simulink model "Lab5p3b"  (R2022a)
settings: Solver=ode3  StartTime=0.0  StopTime=Tmdl  FixedStep=T0/100  RelTol=1e-3
values from neighbouring files (symbols this model uses):
  ob =     [data.mat]
undefined symbols (not defined in the file or in its folder): spl, T0
libraries: fl_lib x22, nesl_utility x18
settings Model: Creator=Egor  LastModifiedBy=vardo

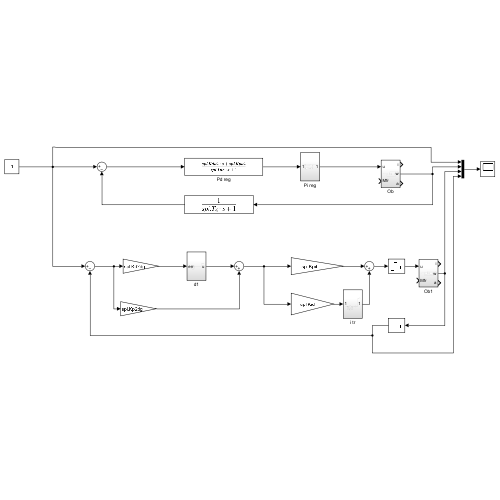
[thumbnail: Simulink's stored preview of the top-level diagram]
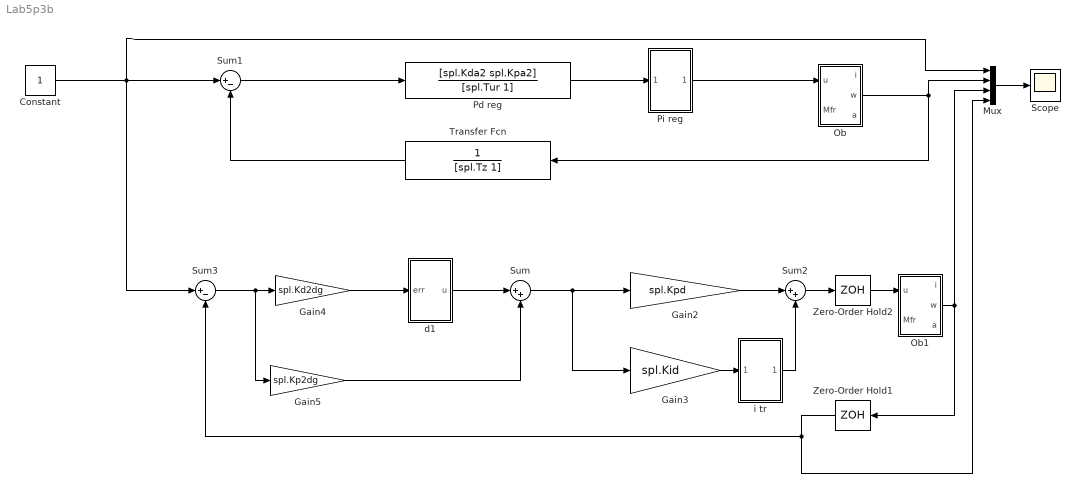
== system Lab5p3b ==
  Constant : Constant
  Gain2 : Gain  Gain=spl.Kpd
  Gain3 : Gain  Gain=spl.Kid
  Gain4 : Gain  Gain=spl.Kd2dg
  Gain5 : Gain  Gain=spl.Kp2dg
  Mux : Mux
  Ob : Subsystem
  Ob1 : Subsystem
  Pd reg : TransferFcn  Numerator=[spl.Kda2 spl.Kpa2]  Denominator=[spl.Tur 1]
  Pi reg : Subsystem
  Scope : Scope
  Sum : Sum  Inputs=|++
  Sum1 : Sum  Inputs=|+-
  Sum2 : Sum  Inputs=|++
  Sum3 : Sum  Inputs=|+-
  Transfer Fcn : TransferFcn  Denominator=[spl.Tz 1]
  Zero-Order Hold1 : ZeroOrderHold  SampleTime=T0
  Zero-Order Hold2 : ZeroOrderHold  SampleTime=T0
  d1 : Subsystem
  i tr : Subsystem
  wires:
  Mux/1 -> Scope/1
  Sum2/1 -> Zero-Order Hold2/1
  i tr/1(Out1) -> Sum2/2
  Gain2/1 -> Sum2/1
  Constant/1 -> Sum3/1, Mux/1, Sum1/1
  Ob1/2(w) -> Mux/3, Zero-Order Hold1/1
  Gain3/1 -> i tr/1(In1)
  Zero-Order Hold2/1 -> Ob1/1(u)
  Zero-Order Hold1/1 -> Mux/4, Sum3/2
  Ob/2(w) -> Transfer Fcn/1, Mux/2
  Sum1/1 -> Pd reg/1
  Pi reg/1(Out1) -> Ob/1(u)
  Pd reg/1 -> Pi reg/1(In1)
  d1/1(u) -> Sum/1
  Gain5/1 -> Sum/2
  Sum3/1 -> Gain5/1, Gain4/1
  Gain4/1 -> d1/1(err)
  Sum/1 -> Gain3/1, Gain2/1
  Transfer Fcn/1 -> Sum1/2

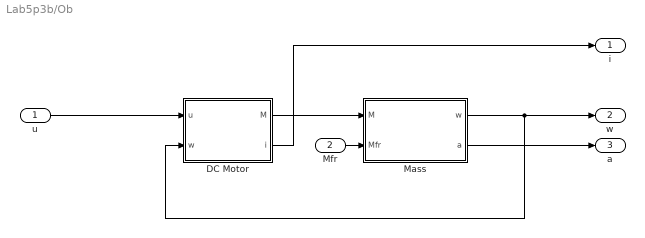
== system Lab5p3b/Ob ==
  u : Inport
  Mfr : Inport  Port=2
  DC Motor : Subsystem
  Mass : Subsystem
  i : Outport
  w : Outport  Port=2
  a : Outport  Port=3
  wires:
  Mass/2(a) -> a/1
  u/1 -> DC Motor/1(u)
  Mass/1(w) -> w/1, DC Motor/2(w)
  DC Motor/1(M) -> Mass/1(M)
  Mfr/1 -> Mass/2(Mfr)
  DC Motor/2(i) -> i/1

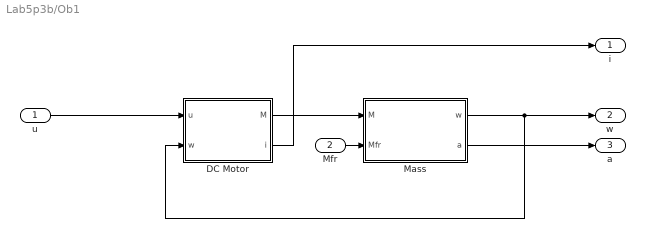
== system Lab5p3b/Ob1 ==
  u : Inport
  Mfr : Inport  Port=2
  DC Motor : Subsystem
  Mass : Subsystem
  i : Outport
  w : Outport  Port=2
  a : Outport  Port=3
  wires:
  Mass/2(a) -> a/1
  u/1 -> DC Motor/1(u)
  Mass/1(w) -> w/1, DC Motor/2(w)
  DC Motor/1(M) -> Mass/1(M)
  Mfr/1 -> Mass/2(Mfr)
  DC Motor/2(i) -> i/1

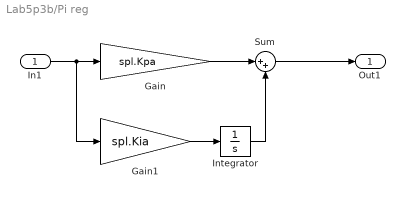
== system Lab5p3b/Pi reg ==
  In1 : Inport
  Gain : Gain  Gain=spl.Kpa
  Gain1 : Gain  Gain=spl.Kia
  Integrator : Integrator
  Sum : Sum  Inputs=|++
  Out1 : Outport
  wires:
  Gain1/1 -> Integrator/1
  In1/1 -> Gain1/1, Gain/1
  Integrator/1 -> Sum/2
  Gain/1 -> Sum/1
  Sum/1 -> Out1/1

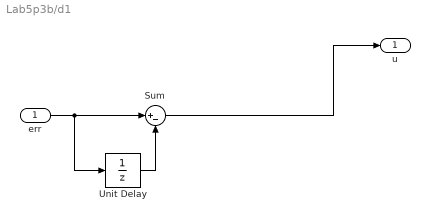
== system Lab5p3b/d1 ==
  err : Inport
  Sum : Sum  Inputs=|+-
  Unit Delay : UnitDelay  SampleTime=T0  HasFrameUpgradeWarning=on
  u : Outport
  wires:
  err/1 -> Unit Delay/1, Sum/1
  Unit Delay/1 -> Sum/2
  Sum/1 -> u/1

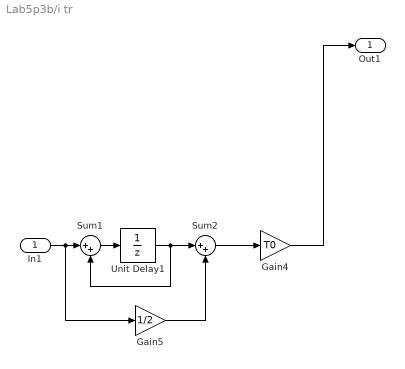
== system Lab5p3b/i tr ==
  In1 : Inport
  Gain4 : Gain  Gain=T0
  Gain5 : Gain  Gain=1/2
  Sum1 : Sum  Inputs=|++
  Sum2 : Sum  Inputs=|++
  Unit Delay1 : UnitDelay  SampleTime=-1  HasFrameUpgradeWarning=on
  Out1 : Outport
  wires:
  In1/1 -> Gain5/1, Sum1/1
  Sum1/1 -> Unit Delay1/1
  Gain5/1 -> Sum2/2
  Gain4/1 -> Out1/1
  Unit Delay1/1 -> Sum2/1, Sum1/2
  Sum2/1 -> Gain4/1

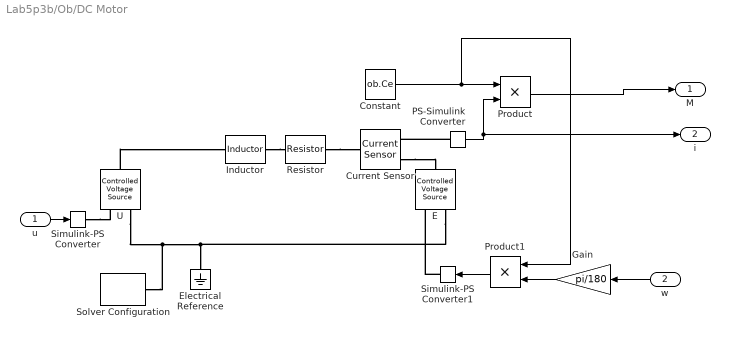
== system Lab5p3b/Ob/DC Motor ==
  u : Inport
  w : Inport  Port=2
  Constant : Constant  Value=ob.Ce
  Current Sensor : fl_lib/Electrical/Electrical Sensors/Current Sensor
      settings: SourceProductBaseCode=PW,SS,VE
  E : fl_lib/Electrical/Electrical Sources/Controlled Voltage Source
      settings: SourceProductBaseCode=PW,SS,VE
  Electrical Reference : fl_lib/Electrical/Electrical Elements/Electrical Reference
      settings: SourceProductBaseCode=PW,SS,VE
  Gain : Gain  Gain=pi/180
  Inductor : fl_lib/Electrical/Electrical Elements/Inductor  l=ob.L H  r=0 Ohm  g=1e-9 1/Ohm  i_specify=off  i_priority=None  i=0 A  i_nominal_specify=off  i_nominal_unit=A  i_nominal_value=1  v_specify=off  v_priority=None  v=0 V  v_nominal_specify=off  v_nominal_unit=V  v_nominal_value=1  i_L_specify=off  i_L_priority=High  i_L=0 A  i_L_nominal_specify=off  i_L_nominal_unit=A  i_L_nominal_value=1
      settings: SourceProductBaseCode=PW,SS,VE
  PS-Simulink Converter : nesl_utility/PS-Simulink Converter  PhysicalDomain=network_engine_domain  SubClassName=ps_output  LeftPortType=input  RightPortType=output  PseudoPeriodic=off  Frequencies=[]  VectorFormat=inherit  Unit=inherit  AffineConversion=off
      settings: SourceProductBaseCode=SS,PW,VE
  Product : Product
  Product1 : Product
  Resistor : fl_lib/Electrical/Electrical Elements/Resistor  R=ob.R Ohm  i_specify=off  i_priority=None  i=0 A  i_nominal_specify=off  i_nominal_unit=A  i_nominal_value=1  v_specify=off  v_priority=None  v=0 V  v_nominal_specify=off  v_nominal_unit=V  v_nominal_value=1
      settings: SourceProductBaseCode=PW,SS,VE
  Simulink-PS Converter : nesl_utility/Simulink-PS Converter  PhysicalDomain=network_engine_domain  SubClassName=ps_input  LeftPortType=input  RightPortType=output  PseudoPeriodic=off  Frequencies=[]  NoiseDistribution=none  NoiseParameters=[]  Unit=1  AffineConversion=off  FilteringAndDerivatives=provide  SimscapeFilterOrder=1  InputFilterTimeConstant=0.0001  UdotUserProvided=0
      settings: SourceProductBaseCode=SS,PW,VE
  Simulink-PS Converter1 : nesl_utility/Simulink-PS Converter  PhysicalDomain=network_engine_domain  SubClassName=ps_input  LeftPortType=input  RightPortType=output  PseudoPeriodic=off  Frequencies=[]  NoiseDistribution=none  NoiseParameters=[]  Unit=1  AffineConversion=off  FilteringAndDerivatives=provide  SimscapeFilterOrder=1  InputFilterTimeConstant=0.001  UdotUserProvided=0
      settings: SourceProductBaseCode=SS,PW,VE
  Solver Configuration : nesl_utility/Solver Configuration  PhysicalDomain=network_engine_domain  SubClassName=solver  LeftPortType=input  RightPortType=generic  Tones=[]  Harmonics=[]  SimulateNoise=off  Profile=off  UseLocalSampling=off  EnableSwitchedLinearOptims=on  FrequencyDomain=off  UseCCode=off  RelTol=0.001  AbsTol=0.001  MinStep=1e-09  ToWorkspace=off  RevertToSquareIcSolve=off  NumHomotopyIterations=100  PhasorMode=off  PhasorModeNumHarmonics=1  IndexReductionMethod=DerivativeReplacement  DoDC=off  ResidualTolerance=1e-09  UseLocalSolver=off  LocalSolverChoice=NE_BACKWARD_EULER_ADVANCER  LocalSolverSampleTime=0.001  DoFixedCost=off  MaxNonlinIter=3  MaxModeIter=2  ComputeImpulses=off  ImpulseIterations=2  LinearAlgebra=auto  LinearAlgebraNumThread=0  EquationFormulation=NE_TIME_EF  DelaysMemoryBudget=1024  AutomaticFiltering=on  FilteringTimeConstant=0.001  PartitionStorageMethod=AS_NEEDED  PartitionMemoryBudget=1024  PartitionMethod=ROBUST
      settings: SourceProductBaseCode=SS,PW,VE
  U : fl_lib/Electrical/Electrical Sources/Controlled Voltage Source
      settings: SourceProductBaseCode=PW,SS,VE
  M : Outport
  i : Outport  Port=2
  wires:
  PS-Simulink Converter/1 -> i/1, Product/2
  Product1/1 -> Simulink-PS Converter1/1
  Constant/1 -> Product1/1, Product/1
  Product/1 -> M/1
  u/1 -> Simulink-PS Converter/1
  w/1 -> Gain/1
  Gain/1 -> Product1/2
  connections:
  Simulink-PS Converter1/RConn1 -- E/RConn1
  Current Sensor/RConn2 -- E/LConn1
  U/LConn1 -- Inductor/LConn1
  U/RConn2 -- Solver Configuration/RConn1 -- E/RConn2 -- Electrical Reference/LConn1
  Resistor/RConn1 -- Current Sensor/LConn1
  Simulink-PS Converter/RConn1 -- U/RConn1
  PS-Simulink Converter/LConn1 -- Current Sensor/RConn1
  Inductor/RConn1 -- Resistor/LConn1

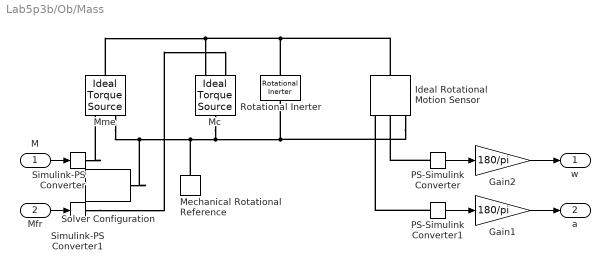
== system Lab5p3b/Ob/Mass ==
  M : Inport
  Mfr : Inport  Port=2
  Gain1 : Gain  Gain=180/pi
  Gain2 : Gain  Gain=180/pi
  Ideal Rotational Motion Sensor : fl_lib/Mechanical/Mechanical Sensors/Ideal Rotational Motion Sensor  wrap_angle=simscape.enum.onoff.off  offset=0 rad
      settings: SourceProductBaseCode=PW,SS,VE
  Mc : fl_lib/Mechanical/Mechanical Sources/Ideal Torque Source
      settings: SourceProductBaseCode=PW,SS,VE
  Mechanical Rotational Reference : fl_lib/Mechanical/Rotational Elements/Mechanical Rotational Reference
      settings: SourceProductBaseCode=PW,SS,VE
  Mme : fl_lib/Mechanical/Mechanical Sources/Ideal Torque Source
      settings: SourceProductBaseCode=PW,SS,VE
  PS-Simulink Converter : nesl_utility/PS-Simulink Converter  PhysicalDomain=network_engine_domain  SubClassName=ps_output  LeftPortType=input  RightPortType=output  PseudoPeriodic=off  Frequencies=[]  VectorFormat=inherit  Unit=inherit  AffineConversion=off
      settings: SourceProductBaseCode=SS,PW,VE
  PS-Simulink Converter1 : nesl_utility/PS-Simulink Converter  PhysicalDomain=network_engine_domain  SubClassName=ps_output  LeftPortType=input  RightPortType=output  PseudoPeriodic=off  Frequencies=[]  VectorFormat=inherit  Unit=inherit  AffineConversion=off
      settings: SourceProductBaseCode=SS,PW,VE
  Rotational Inerter : fl_lib/Mechanical/Rotational Elements/Rotational Inerter  B=ob.J kg*m^2  w_specify=off  w_priority=High  w=0 rad/s  w_nominal_specify=off  w_nominal_unit=rad/s  w_nominal_value=1  t_specify=off  t_priority=None  t=0 N*m  t_nominal_specify=off  t_nominal_unit=N*m  t_nominal_value=1
      settings: SourceProductBaseCode=PW,SS,VE  InternalSimscapePortConfiguration="{\"Bottom\":[],\"Left\":[{\"id\":\"R\",\"label\":\"R\",\"type\":\"foundation.mechanical.rotational.rotational\"}],\"Right\":[{\"id\":\"C\",\"label\":\"C\",\"type\":\"foundation.mechanical.rotational.rotational\"}],\"Top\":[]}"
  Simulink-PS Converter : nesl_utility/Simulink-PS Converter  PhysicalDomain=network_engine_domain  SubClassName=ps_input  LeftPortType=input  RightPortType=output  PseudoPeriodic=off  Frequencies=[]  NoiseDistribution=none  NoiseParameters=[]  Unit=1  AffineConversion=off  FilteringAndDerivatives=provide  SimscapeFilterOrder=1  InputFilterTimeConstant=0.001  UdotUserProvided=0
      settings: SourceProductBaseCode=SS,PW,VE
  Simulink-PS Converter1 : nesl_utility/Simulink-PS Converter  PhysicalDomain=network_engine_domain  SubClassName=ps_input  LeftPortType=input  RightPortType=output  PseudoPeriodic=off  Frequencies=[]  NoiseDistribution=none  NoiseParameters=[]  Unit=1  AffineConversion=off  FilteringAndDerivatives=provide  SimscapeFilterOrder=1  InputFilterTimeConstant=0.001  UdotUserProvided=0
      settings: SourceProductBaseCode=SS,PW,VE
  Solver Configuration : nesl_utility/Solver Configuration  PhysicalDomain=network_engine_domain  SubClassName=solver  LeftPortType=input  RightPortType=generic  Tones=[]  Harmonics=[]  SimulateNoise=off  Profile=off  UseLocalSampling=off  EnableSwitchedLinearOptims=on  FrequencyDomain=off  UseCCode=off  RelTol=0.001  AbsTol=0.001  MinStep=1e-09  ToWorkspace=off  RevertToSquareIcSolve=off  NumHomotopyIterations=100  PhasorMode=off  PhasorModeNumHarmonics=1  IndexReductionMethod=DerivativeReplacement  DoDC=off  ResidualTolerance=1e-09  UseLocalSolver=off  LocalSolverChoice=NE_BACKWARD_EULER_ADVANCER  LocalSolverSampleTime=0.001  DoFixedCost=off  MaxNonlinIter=3  MaxModeIter=2  ComputeImpulses=off  ImpulseIterations=2  LinearAlgebra=auto  LinearAlgebraNumThread=0  EquationFormulation=NE_TIME_EF  DelaysMemoryBudget=1024  AutomaticFiltering=on  FilteringTimeConstant=0.001  PartitionStorageMethod=AS_NEEDED  PartitionMemoryBudget=1024  PartitionMethod=ROBUST
      settings: SourceProductBaseCode=SS,PW,VE
  w : Outport
  a : Outport  Port=2
  wires:
  PS-Simulink Converter/1 -> Gain2/1
  PS-Simulink Converter1/1 -> Gain1/1
  M/1 -> Simulink-PS Converter/1
  Mfr/1 -> Simulink-PS Converter1/1
  Gain2/1 -> w/1
  Gain1/1 -> a/1
  connections:
  Mme/LConn1 -- Ideal Rotational Motion Sensor/LConn1 -- Rotational Inerter/LConn1 -- Mc/RConn2
  Simulink-PS Converter/RConn1 -- Mme/RConn1
  Mme/RConn2 -- Solver Configuration/RConn1 -- Mechanical Rotational Reference/LConn1 -- Mc/LConn1 -- Ideal Rotational Motion Sensor/RConn1 -- Rotational Inerter/RConn1
  Simulink-PS Converter1/RConn1 -- Mc/RConn1
  PS-Simulink Converter1/LConn1 -- Ideal Rotational Motion Sensor/RConn3
  PS-Simulink Converter/LConn1 -- Ideal Rotational Motion Sensor/RConn2

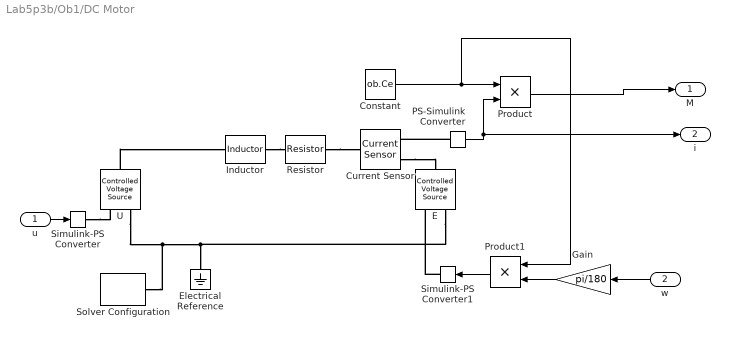
== system Lab5p3b/Ob1/DC Motor ==
  u : Inport
  w : Inport  Port=2
  Constant : Constant  Value=ob.Ce
  Current Sensor : fl_lib/Electrical/Electrical Sensors/Current Sensor
      settings: SourceProductBaseCode=PW,SS,VE
  E : fl_lib/Electrical/Electrical Sources/Controlled Voltage Source
      settings: SourceProductBaseCode=PW,SS,VE
  Electrical Reference : fl_lib/Electrical/Electrical Elements/Electrical Reference
      settings: SourceProductBaseCode=PW,SS,VE
  Gain : Gain  Gain=pi/180
  Inductor : fl_lib/Electrical/Electrical Elements/Inductor  l=ob.L H  r=0 Ohm  g=1e-9 1/Ohm  i_specify=off  i_priority=None  i=0 A  i_nominal_specify=off  i_nominal_unit=A  i_nominal_value=1  v_specify=off  v_priority=None  v=0 V  v_nominal_specify=off  v_nominal_unit=V  v_nominal_value=1  i_L_specify=off  i_L_priority=High  i_L=0 A  i_L_nominal_specify=off  i_L_nominal_unit=A  i_L_nominal_value=1
      settings: SourceProductBaseCode=PW,SS,VE
  PS-Simulink Converter : nesl_utility/PS-Simulink Converter  PhysicalDomain=network_engine_domain  SubClassName=ps_output  LeftPortType=input  RightPortType=output  PseudoPeriodic=off  Frequencies=[]  VectorFormat=inherit  Unit=inherit  AffineConversion=off
      settings: SourceProductBaseCode=SS,PW,VE
  Product : Product
  Product1 : Product
  Resistor : fl_lib/Electrical/Electrical Elements/Resistor  R=ob.R Ohm  i_specify=off  i_priority=None  i=0 A  i_nominal_specify=off  i_nominal_unit=A  i_nominal_value=1  v_specify=off  v_priority=None  v=0 V  v_nominal_specify=off  v_nominal_unit=V  v_nominal_value=1
      settings: SourceProductBaseCode=PW,SS,VE
  Simulink-PS Converter : nesl_utility/Simulink-PS Converter  PhysicalDomain=network_engine_domain  SubClassName=ps_input  LeftPortType=input  RightPortType=output  PseudoPeriodic=off  Frequencies=[]  NoiseDistribution=none  NoiseParameters=[]  Unit=1  AffineConversion=off  FilteringAndDerivatives=provide  SimscapeFilterOrder=1  InputFilterTimeConstant=0.0001  UdotUserProvided=0
      settings: SourceProductBaseCode=SS,PW,VE
  Simulink-PS Converter1 : nesl_utility/Simulink-PS Converter  PhysicalDomain=network_engine_domain  SubClassName=ps_input  LeftPortType=input  RightPortType=output  PseudoPeriodic=off  Frequencies=[]  NoiseDistribution=none  NoiseParameters=[]  Unit=1  AffineConversion=off  FilteringAndDerivatives=provide  SimscapeFilterOrder=1  InputFilterTimeConstant=0.001  UdotUserProvided=0
      settings: SourceProductBaseCode=SS,PW,VE
  Solver Configuration : nesl_utility/Solver Configuration  PhysicalDomain=network_engine_domain  SubClassName=solver  LeftPortType=input  RightPortType=generic  Tones=[]  Harmonics=[]  SimulateNoise=off  Profile=off  UseLocalSampling=off  EnableSwitchedLinearOptims=on  FrequencyDomain=off  UseCCode=off  RelTol=0.001  AbsTol=0.001  MinStep=1e-09  ToWorkspace=off  RevertToSquareIcSolve=off  NumHomotopyIterations=100  PhasorMode=off  PhasorModeNumHarmonics=1  IndexReductionMethod=DerivativeReplacement  DoDC=off  ResidualTolerance=1e-09  UseLocalSolver=off  LocalSolverChoice=NE_BACKWARD_EULER_ADVANCER  LocalSolverSampleTime=0.001  DoFixedCost=off  MaxNonlinIter=3  MaxModeIter=2  ComputeImpulses=off  ImpulseIterations=2  LinearAlgebra=auto  LinearAlgebraNumThread=0  EquationFormulation=NE_TIME_EF  DelaysMemoryBudget=1024  AutomaticFiltering=on  FilteringTimeConstant=0.001  PartitionStorageMethod=AS_NEEDED  PartitionMemoryBudget=1024  PartitionMethod=ROBUST
      settings: SourceProductBaseCode=SS,PW,VE
  U : fl_lib/Electrical/Electrical Sources/Controlled Voltage Source
      settings: SourceProductBaseCode=PW,SS,VE
  M : Outport
  i : Outport  Port=2
  wires:
  PS-Simulink Converter/1 -> i/1, Product/2
  Product1/1 -> Simulink-PS Converter1/1
  Constant/1 -> Product1/1, Product/1
  Product/1 -> M/1
  u/1 -> Simulink-PS Converter/1
  w/1 -> Gain/1
  Gain/1 -> Product1/2
  connections:
  Simulink-PS Converter1/RConn1 -- E/RConn1
  Current Sensor/RConn2 -- E/LConn1
  U/LConn1 -- Inductor/LConn1
  U/RConn2 -- Solver Configuration/RConn1 -- E/RConn2 -- Electrical Reference/LConn1
  Resistor/RConn1 -- Current Sensor/LConn1
  Simulink-PS Converter/RConn1 -- U/RConn1
  PS-Simulink Converter/LConn1 -- Current Sensor/RConn1
  Inductor/RConn1 -- Resistor/LConn1

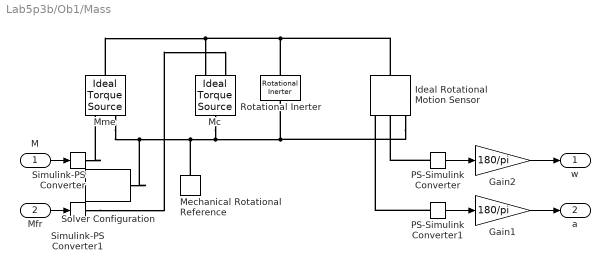
== system Lab5p3b/Ob1/Mass ==
  M : Inport
  Mfr : Inport  Port=2
  Gain1 : Gain  Gain=180/pi
  Gain2 : Gain  Gain=180/pi
  Ideal Rotational Motion Sensor : fl_lib/Mechanical/Mechanical Sensors/Ideal Rotational Motion Sensor  wrap_angle=simscape.enum.onoff.off  offset=0 rad
      settings: SourceProductBaseCode=PW,SS,VE
  Mc : fl_lib/Mechanical/Mechanical Sources/Ideal Torque Source
      settings: SourceProductBaseCode=PW,SS,VE
  Mechanical Rotational Reference : fl_lib/Mechanical/Rotational Elements/Mechanical Rotational Reference
      settings: SourceProductBaseCode=PW,SS,VE
  Mme : fl_lib/Mechanical/Mechanical Sources/Ideal Torque Source
      settings: SourceProductBaseCode=PW,SS,VE
  PS-Simulink Converter : nesl_utility/PS-Simulink Converter  PhysicalDomain=network_engine_domain  SubClassName=ps_output  LeftPortType=input  RightPortType=output  PseudoPeriodic=off  Frequencies=[]  VectorFormat=inherit  Unit=inherit  AffineConversion=off
      settings: SourceProductBaseCode=SS,PW,VE
  PS-Simulink Converter1 : nesl_utility/PS-Simulink Converter  PhysicalDomain=network_engine_domain  SubClassName=ps_output  LeftPortType=input  RightPortType=output  PseudoPeriodic=off  Frequencies=[]  VectorFormat=inherit  Unit=inherit  AffineConversion=off
      settings: SourceProductBaseCode=SS,PW,VE
  Rotational Inerter : fl_lib/Mechanical/Rotational Elements/Rotational Inerter  B=ob.J kg*m^2  w_specify=off  w_priority=High  w=0 rad/s  w_nominal_specify=off  w_nominal_unit=rad/s  w_nominal_value=1  t_specify=off  t_priority=None  t=0 N*m  t_nominal_specify=off  t_nominal_unit=N*m  t_nominal_value=1
      settings: SourceProductBaseCode=PW,SS,VE  InternalSimscapePortConfiguration="{\"Bottom\":[],\"Left\":[{\"id\":\"R\",\"label\":\"R\",\"type\":\"foundation.mechanical.rotational.rotational\"}],\"Right\":[{\"id\":\"C\",\"label\":\"C\",\"type\":\"foundation.mechanical.rotational.rotational\"}],\"Top\":[]}"
  Simulink-PS Converter : nesl_utility/Simulink-PS Converter  PhysicalDomain=network_engine_domain  SubClassName=ps_input  LeftPortType=input  RightPortType=output  PseudoPeriodic=off  Frequencies=[]  NoiseDistribution=none  NoiseParameters=[]  Unit=1  AffineConversion=off  FilteringAndDerivatives=provide  SimscapeFilterOrder=1  InputFilterTimeConstant=0.001  UdotUserProvided=0
      settings: SourceProductBaseCode=SS,PW,VE
  Simulink-PS Converter1 : nesl_utility/Simulink-PS Converter  PhysicalDomain=network_engine_domain  SubClassName=ps_input  LeftPortType=input  RightPortType=output  PseudoPeriodic=off  Frequencies=[]  NoiseDistribution=none  NoiseParameters=[]  Unit=1  AffineConversion=off  FilteringAndDerivatives=provide  SimscapeFilterOrder=1  InputFilterTimeConstant=0.001  UdotUserProvided=0
      settings: SourceProductBaseCode=SS,PW,VE
  Solver Configuration : nesl_utility/Solver Configuration  PhysicalDomain=network_engine_domain  SubClassName=solver  LeftPortType=input  RightPortType=generic  Tones=[]  Harmonics=[]  SimulateNoise=off  Profile=off  UseLocalSampling=off  EnableSwitchedLinearOptims=on  FrequencyDomain=off  UseCCode=off  RelTol=0.001  AbsTol=0.001  MinStep=1e-09  ToWorkspace=off  RevertToSquareIcSolve=off  NumHomotopyIterations=100  PhasorMode=off  PhasorModeNumHarmonics=1  IndexReductionMethod=DerivativeReplacement  DoDC=off  ResidualTolerance=1e-09  UseLocalSolver=off  LocalSolverChoice=NE_BACKWARD_EULER_ADVANCER  LocalSolverSampleTime=0.001  DoFixedCost=off  MaxNonlinIter=3  MaxModeIter=2  ComputeImpulses=off  ImpulseIterations=2  LinearAlgebra=auto  LinearAlgebraNumThread=0  EquationFormulation=NE_TIME_EF  DelaysMemoryBudget=1024  AutomaticFiltering=on  FilteringTimeConstant=0.001  PartitionStorageMethod=AS_NEEDED  PartitionMemoryBudget=1024  PartitionMethod=ROBUST
      settings: SourceProductBaseCode=SS,PW,VE
  w : Outport
  a : Outport  Port=2
  wires:
  PS-Simulink Converter/1 -> Gain2/1
  PS-Simulink Converter1/1 -> Gain1/1
  M/1 -> Simulink-PS Converter/1
  Mfr/1 -> Simulink-PS Converter1/1
  Gain2/1 -> w/1
  Gain1/1 -> a/1
  connections:
  Mme/LConn1 -- Ideal Rotational Motion Sensor/LConn1 -- Rotational Inerter/LConn1 -- Mc/RConn2
  Simulink-PS Converter/RConn1 -- Mme/RConn1
  Mme/RConn2 -- Solver Configuration/RConn1 -- Mechanical Rotational Reference/LConn1 -- Mc/LConn1 -- Ideal Rotational Motion Sensor/RConn1 -- Rotational Inerter/RConn1
  Simulink-PS Converter1/RConn1 -- Mc/RConn1
  PS-Simulink Converter1/LConn1 -- Ideal Rotational Motion Sensor/RConn3
  PS-Simulink Converter/LConn1 -- Ideal Rotational Motion Sensor/RConn2
